simulink model "SelectionDepart"  (R2025a)
settings: Solver=VariableStepAuto  StartTime=0.0  StopTime=0.1  RelTol=1e-3
values from neighbouring files (symbols this model uses):
  fba = (Val + 18) - fi    (= 888)    [Variables.m]
  fbn = (Val2 + 47.5) - fi    (= 920)    [Variables.m]
  m = 8    [Variables.m]
  offseta = 33    [Variables.m]
  offsetn = 100    [Variables.m]
  type = 0    [Variables.m]
undefined symbols (not defined in the file or in its folder): n
libraries: dspfdesign x11, dspsigops x1, dspobslib x1
settings Model: Creator=roys2121  LastModifiedBy=francoisdesautels
settings DebuggingCC: UnconnectedInputMsg=warning  UnconnectedOutputMsg=warning  UnconnectedLineMsg=warning
settings ModelReferenceCC: EnableRefExpFcnMdlSchedulingChecks=on
settings RTWCC: GPUComputeCapability=3.5  DLArmComputeVersion=19.05

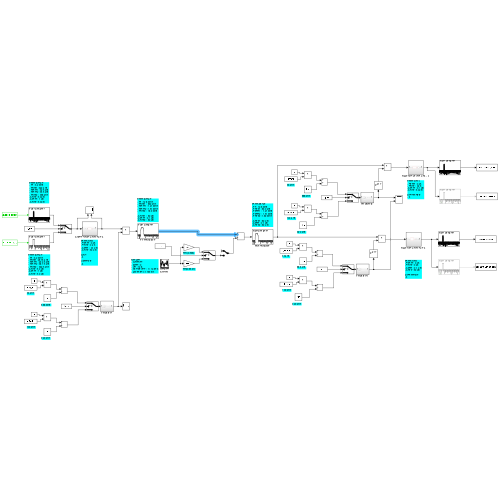
[thumbnail: Simulink's stored preview of the top-level diagram]
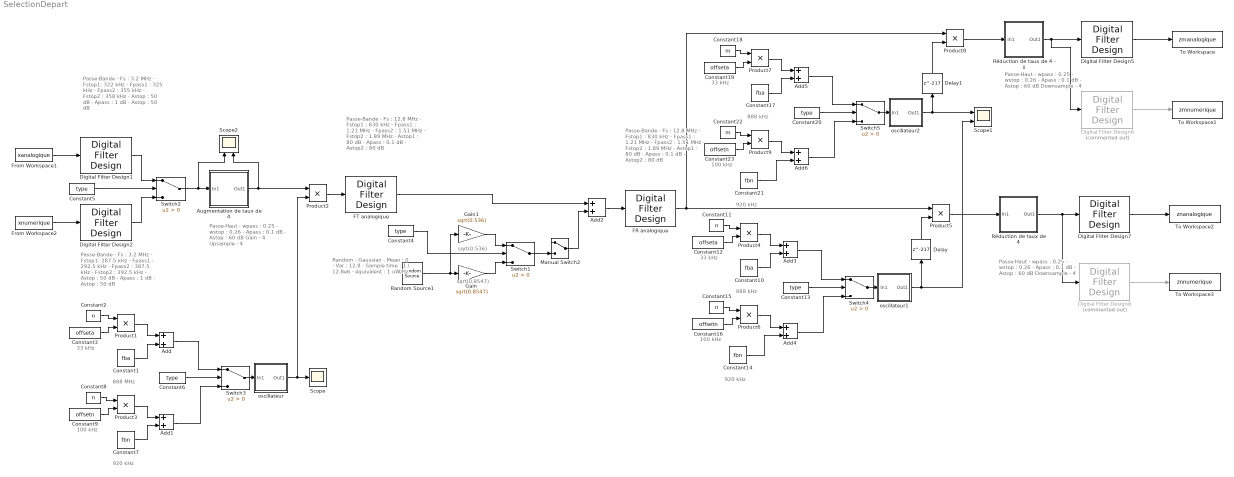
== system SelectionDepart ==
  note: 888 MHz
  note: 33 kHz
  note: 100 kHz
  note: 920 kHz
  note: Passe-Bande
      | - Fs : 3.2 MHz
      | - Fstop1: 322 kHz
      | - Fpass1 : 325 kHz
      | - Fpass2 : 355 kHz
      | - Fstop2 : 358 kHz
      | - Astop : 50 dB
      | - Apass : 1 dB
      | - Astop : 50 dB
  note: Passe-Bande
      | - Fs : 3.2 MHz
      | - Fstop1: 287.5 kHz
      | - Fpass1 : 292.5 kHz
      | - Fpass2 : 387.5 kHz
      | - Fstop2 : 392.5 kHz
      | - Astop : 50 dB
      | - Apass : 1 dB
      | - Astop : 50 dB
  note: Passe-Haut
      | - wpass : 0.25
      | - wstop : 0.26
      | - Apass : 0.1 dB
      | - Astop : 60 dB
      |
      | Gain
      | - 4
      |
      | Upsample
      | - 4
  note: Passe-Haut
      | - wpass : 0.25
      | - wstop : 0.26
      | - Apass : 0.1 dB
      | - Astop : 60 dB
      |
      | Downsample
      | - 4
  note: Passe-Haut
      | - wpass : 0.25
      | - wstop : 0.26
      | - Apass : 0.1 dB
      | - Astop : 60 dB
      |
      | Downsample
      | - 4
  note: Passe-Bande
      | - Fs : 12.8 MHz
      | - Fstop1 : 830 kHz
      | - Fpass1 : 1.21 MHz
      | - Fpass2 : 1.51 MHz
      | - Fstop2 : 1.89 MHz
      |
      | - Astop1 : 80 dB
      | - Apass : 0.1 dB
      | - Astop2 : 80 dB
  note: Passe-Bande
      | - Fs : 12.8 MHz
      | - Fstop1 : 830 kHz
      | - Fpass1 : 1.21 MHz
      | - Fpass2 : 1.51 MHz
      | - Fstop2 : 1.89 MHz
      |
      | - Astop1 : 80 dB
      | - Apass : 0.1 dB
      | - Astop2 : 80 dB
  note: Random
      | - Gaussian
      | - Mean : 0
      | - Var : 12.8
      | - Sample time : 1 / 12.8e6
      | - équivalent : 1 uW/Hz
  note: sqrt(0.536)
  note: sqrt(0.8547)
  note: 33 kHz
  note: 888 kHz
  note: 920 kHz
  note: 100 kHz
  note: 33 kHz
  note: 888 kHz
  note: 920 kHz
  note: 100 kHz
  Add{,1..6} (7 alike) : Sum
  Augmentation de taux de 4 : Subsystem
  Constant1 : Constant  Value=fba
  Constant10 : Constant  Value=fba
  Constant{2,8,11,15} (4 alike) : Constant  Value=n
  Constant12 : Constant  Value=offseta
  Constant{4..6,13,20} (5 alike) : Constant  Value=type
  Constant14 : Constant  Value=fbn
  Constant16 : Constant  Value=offsetn
  Constant17 : Constant  Value=fba
  Constant18 : Constant  Value=m
  Constant19 : Constant  Value=offseta
  Constant21 : Constant  Value=fbn
  Constant22 : Constant  Value=m
  Constant23 : Constant  Value=offsetn
  Constant3 : Constant  Value=offseta
  Constant7 : Constant  Value=fbn
  Constant9 : Constant  Value=offsetn
  Delay : Delay  DelayLength=217  InitialCondition=0
  Delay1 : Delay  DelayLength=217  InitialCondition=0
  Digital Filter Design{1..2,5,7} (4 alike) : dspfdesign/Digital Filter Design  mwdsp_browser_bugfix_var=off
  Digital Filter Design6 : dspfdesign/Digital Filter Design  Commented=on  mwdsp_browser_bugfix_var=off
  Digital Filter Design8 : dspfdesign/Digital Filter Design  Commented=on  mwdsp_browser_bugfix_var=off
  FR analogique : dspfdesign/Digital Filter Design  mwdsp_browser_bugfix_var=off
  FT analogique : dspfdesign/Digital Filter Design  mwdsp_browser_bugfix_var=off
  From Workspace1 : FromWorkspace  VariableName=xanalogique  SampleTime=1/3.2e6  Interpolate=off  ZeroCross=off  OutputAfterFinalValue=Setting to zero
  From Workspace2 : FromWorkspace  VariableName=xnumerique  SampleTime=1/3.2e6  Interpolate=off  OutputAfterFinalValue=Setting to zero
  Gain : Gain  Gain=sqrt(0.8547)
  Gain1 : Gain  Gain=sqrt(0.536)
  Manual Switch2 : ManualSwitch
  Product{1..9} (9 alike) : Product
  Random Source1 : dspobslib/Random Source  SrcType=Gaussian  NormMethod=Ziggurat  CltLength=12  MinVal=0  MaxVal=1  MeanVal=0  VarVal=12.8  RepMode=Not repeatable  rawSeed=1  IsInherit=off  SampMode=Discrete  SampTime=1/12.8e6  SampFrame=1  DataType=Double  OutComplex=Real  OutputFrames=off
  Réduction de taux de 4 : Subsystem
  Réduction de taux de 4 - ii : Subsystem
  Scope : Scope
      settings: ActiveDisplayYMinimum=-1.25  ActiveDisplayYMaximum=1.25
  Scope1 : Scope  NumInputPorts=2
      settings: ActiveDisplayYMinimum=-1.25  ActiveDisplayYMaximum=1.25
  Scope2 : Scope  NumInputPorts=2
      settings: ActiveDisplayYMinimum=-5.9294378460727044  ActiveDisplayYMaximum=5.9271411947500114  DataLoggingVariableName=ScopeData2
  Switch{1..5} (5 alike) : Switch  Criteria=u2 > Threshold  SaturateOnIntegerOverflow=off  InputSameDT=off
  To Workspace : ToWorkspace  VariableName=zmanalogique  SaveFormat=Timeseries  SampleTime=-1
      settings: Save2DSignal=2-D array (concatenate along first dimension)
  To Workspace1 : ToWorkspace  VariableName=zmnumerique  SaveFormat=Timeseries  SampleTime=-1
      settings: Save2DSignal=2-D array (concatenate along first dimension)
  To Workspace2 : ToWorkspace  VariableName=znanalogique  SaveFormat=Timeseries  SampleTime=-1
      settings: Save2DSignal=2-D array (concatenate along first dimension)
  To Workspace3 : ToWorkspace  VariableName=znnumerique  SaveFormat=Timeseries  SampleTime=-1
      settings: Save2DSignal=2-D array (concatenate along first dimension)
  oscillateur : Subsystem
  oscillateur1 : Subsystem
  oscillateur2 : Subsystem
  wires:
  From Workspace1/1 -> Digital Filter Design1/1
  From Workspace2/1 -> Digital Filter Design2/1
  oscillateur/1(Out1) -> Product2/2, Scope/1
  Constant2/1 -> Product1/1
  Constant3/1 -> Product1/2
  Constant1/1 -> Add/2
  Product1/1 -> Add/1
  Manual Switch2/1 -> Add2/2
  FT analogique/1 -> Add2/1
  Constant4/1 -> Switch1/2
  Switch1/1 -> Manual Switch2/2
  Random Source1/1 -> Gain1/1, Gain/1
  Gain/1 -> Switch1/3
  Gain1/1 -> Switch1/1
  Augmentation de taux de 4/1(Out1) -> Product2/1, Scope2/2
  Digital Filter Design2/1 -> Switch2/3
  Digital Filter Design1/1 -> Switch2/1
  Switch2/1 -> Augmentation de taux de 4/1(In1), Scope2/1
  Constant5/1 -> Switch2/2
  Constant6/1 -> Switch3/2
  Switch3/1 -> oscillateur/1(In1)
  Add/1 -> Switch3/1
  Constant8/1 -> Product3/1
  Constant9/1 -> Product3/2
  Constant7/1 -> Add1/2
  Product3/1 -> Add1/1
  Add1/1 -> Switch3/3
  Constant11/1 -> Product4/1
  Constant15/1 -> Product6/1
  Constant12/1 -> Product4/2
  Product4/1 -> Add3/1
  oscillateur1/1(Out1) -> Delay/1, Scope1/2
  Constant16/1 -> Product6/2
  Constant13/1 -> Switch4/2
  Add4/1 -> Switch4/3
  Constant14/1 -> Add4/2
  Constant10/1 -> Add3/2
  Add3/1 -> Switch4/1
  Product6/1 -> Add4/1
  Switch4/1 -> oscillateur1/1(In1)
  FR analogique/1 -> Product8/1, Product5/1
  Delay/1 -> Product5/2
  Product9/1 -> Add6/1
  Add5/1 -> Switch5/1
  Delay1/1 -> Product8/2
  Constant21/1 -> Add6/2
  Constant19/1 -> Product7/2
  Add6/1 -> Switch5/3
  Switch5/1 -> oscillateur2/1(In1)
  Constant23/1 -> Product9/2
  Product7/1 -> Add5/1
  oscillateur2/1(Out1) -> Delay1/1, Scope1/1
  Constant20/1 -> Switch5/2
  Constant17/1 -> Add5/2
  Constant18/1 -> Product7/1
  Constant22/1 -> Product9/1
  Réduction de taux de 4 - ii/1(Out1) -> Digital Filter Design6/1, Digital Filter Design5/1
  Réduction de taux de 4/1(Out1) -> Digital Filter Design8/1, Digital Filter Design7/1
  Digital Filter Design7/1 -> To Workspace2/1
  Digital Filter Design8/1 -> To Workspace3/1
  Digital Filter Design5/1 -> To Workspace/1
  Digital Filter Design6/1 -> To Workspace1/1
  Product8/1 -> Réduction de taux de 4 - ii/1(In1)
  Product5/1 -> Réduction de taux de 4/1(In1)
  Product2/1 -> FT analogique/1
  Add2/1 -> FR analogique/1

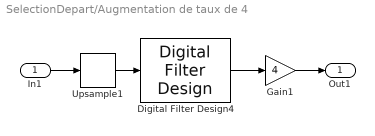
== system SelectionDepart/Augmentation de taux de 4 ==
  In1 : Inport
  Digital Filter Design4 : dspfdesign/Digital Filter Design  mwdsp_browser_bugfix_var=off
  Gain1 : Gain  Gain=4
  Upsample1 : dspsigops/Upsample  FactorSource=Dialog parameter  N=4  Nmax=16  phase=0  RateOptions=Allow multirate processing  ic=0  mode=Unused parameter value
  Out1 : Outport
  wires:
  Upsample1/1 -> Digital Filter Design4/1
  Gain1/1 -> Out1/1
  Digital Filter Design4/1 -> Gain1/1
  In1/1 -> Upsample1/1

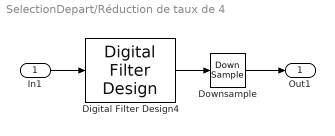
== system SelectionDepart/Réduction de taux de 4 ==
  In1 : Inport
  Digital Filter Design4 : dspfdesign/Digital Filter Design  mwdsp_browser_bugfix_var=off
  Downsample : DownSample  N=4  RateOptions=Allow multirate processing
  Out1 : Outport
  wires:
  In1/1 -> Digital Filter Design4/1
  Digital Filter Design4/1 -> Downsample/1
  Downsample/1 -> Out1/1

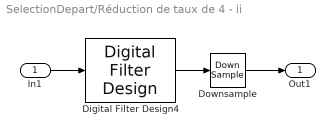
== system SelectionDepart/Réduction de taux de 4 - ii ==
  In1 : Inport
  Digital Filter Design4 : dspfdesign/Digital Filter Design  mwdsp_browser_bugfix_var=off
  Downsample : DownSample  N=4  RateOptions=Allow multirate processing
  Out1 : Outport
  wires:
  Downsample/1 -> Out1/1
  In1/1 -> Digital Filter Design4/1
  Digital Filter Design4/1 -> Downsample/1

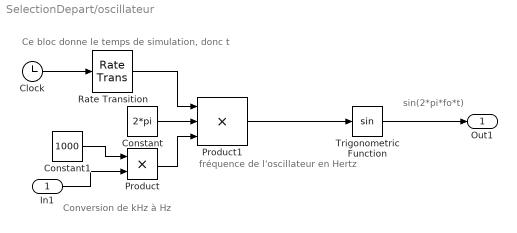
== system SelectionDepart/oscillateur ==
  note: sin(2*pi*fo*t)
  note: Conversion de kHz à Hz
  note: Ce bloc donne le temps de simulation, donc t
  note: fréquence de l'oscillateur en Hertz
  In1 : Inport
  Clock : Clock
  Constant : Constant  Value=2*pi
  Constant1 : Constant  Value=1000
  Product : Product
  Product1 : Product  Inputs=3
  Rate Transition : RateTransition  OutPortSampleTime=1/12.8e6
  Trigonometric Function : Trigonometry
  Out1 : Outport
  wires:
  Trigonometric Function/1 -> Out1/1
  Product1/1 -> Trigonometric Function/1
  Constant/1 -> Product1/2
  Product/1 -> Product1/3
  In1/1 -> Product/2
  Constant1/1 -> Product/1
  Clock/1 -> Rate Transition/1
  Rate Transition/1 -> Product1/1

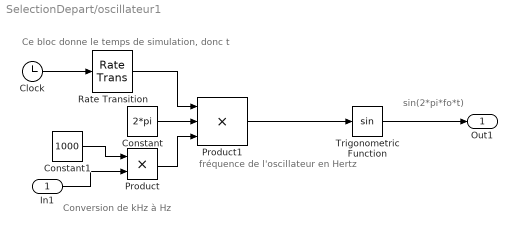
== system SelectionDepart/oscillateur1 ==
  note: sin(2*pi*fo*t)
  note: Conversion de kHz à Hz
  note: Ce bloc donne le temps de simulation, donc t
  note: fréquence de l'oscillateur en Hertz
  In1 : Inport
  Clock : Clock
  Constant : Constant  Value=2*pi
  Constant1 : Constant  Value=1000
  Product : Product
  Product1 : Product  Inputs=3
  Rate Transition : RateTransition  OutPortSampleTime=1/12.8e6
  Trigonometric Function : Trigonometry
  Out1 : Outport
  wires:
  Trigonometric Function/1 -> Out1/1
  Product1/1 -> Trigonometric Function/1
  Constant/1 -> Product1/2
  Product/1 -> Product1/3
  In1/1 -> Product/2
  Constant1/1 -> Product/1
  Clock/1 -> Rate Transition/1
  Rate Transition/1 -> Product1/1

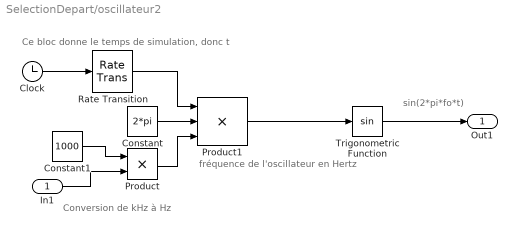
== system SelectionDepart/oscillateur2 ==
  note: sin(2*pi*fo*t)
  note: Conversion de kHz à Hz
  note: Ce bloc donne le temps de simulation, donc t
  note: fréquence de l'oscillateur en Hertz
  In1 : Inport
  Clock : Clock
  Constant : Constant  Value=2*pi
  Constant1 : Constant  Value=1000
  Product : Product
  Product1 : Product  Inputs=3
  Rate Transition : RateTransition  OutPortSampleTime=1/12.8e6
  Trigonometric Function : Trigonometry
  Out1 : Outport
  wires:
  Trigonometric Function/1 -> Out1/1
  Product1/1 -> Trigonometric Function/1
  Constant/1 -> Product1/2
  Product/1 -> Product1/3
  In1/1 -> Product/2
  Constant1/1 -> Product/1
  Clock/1 -> Rate Transition/1
  Rate Transition/1 -> Product1/1
